simulink model "L03"  (R2020b)
settings: Solver=FixedStepDiscrete  StartTime=0.0  StopTime=50.0  FixedStep=0.01  RelTol=1e-3
undefined symbols (not defined in the file): sigbuilder_block
settings Model: Creator=Nic  LastModifiedBy=Nic

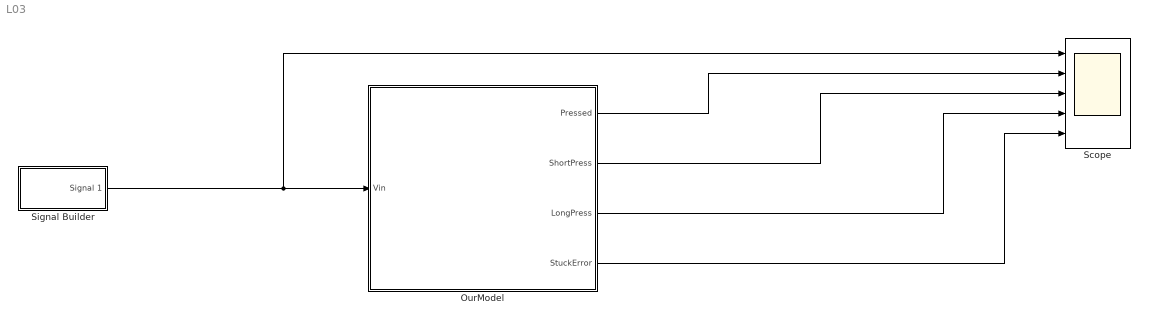
== system L03 ==
  OurModel : Subsystem
  Scope : Scope  NumInputPorts=5
  Signal Builder : Subsystem  Tag=STV Subsys  LoadFcn=sigbuilder_block('load',[173.4 138 748.8 400.2 ]);  StartFcn=sigbuilder_block('start');  StopFcn=sigbuilder_block('stop');  ClipboardFcn=sigbuilder_block('clipboard');  mask(Sigbuilder block){tuvar=[0:10]}
      mask help: Simulink:masks:SigbuilderBlock_MD
      mask init:
      | if ~strcmp(get_param(bdroot(gcbh),'SimulationStatus'),'stopped') tuvar = sigbuilder_block('maskInit'); end
      settings: CopyFcn=sigbuilder_block('copy');  DeleteFcn=sigbuilder_block('delete');  ModelCloseFcn=sigbuilder_block('modelClose');  PreSaveFcn=sigbuilder_block('preSave');  PauseFcn=sigbuilder_block('pause');  ContinueFcn=sigbuilder_block('continue');  NameChangeFcn=sigbuilder_block('namechange');  OpenFcn=sigbuilder_block('open',[173.4 138 550.8 400.2 ]);  CloseFcn=sigbuilder_block('close');
      mask Display: plot(0, 0, 100, 100,[2, 2, 32, 32, 2], [68, 8, 8, 68, 68],[32, 2], [38, 38], [32, 19, 2],[53, 60, 44], [32, 17, 17, 2],[16, 16, 31, 31]);txt = getActiveGroup(gcbh);text(2, 100, txt,'verticalAlignment', 'top');
  wires:
  Signal Builder/1(Signal 1) -> Scope/1, OurModel/1(Vin)
  OurModel/1(Pressed) -> Scope/2
  OurModel/2(ShortPress) -> Scope/3
  OurModel/3(LongPress) -> Scope/4
  OurModel/4(StuckError) -> Scope/5

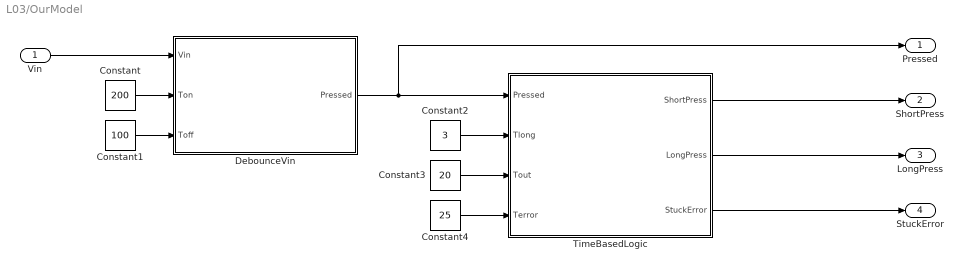
== system L03/OurModel ==
  Vin : Inport
  Constant : Constant  Value=200
  Constant1 : Constant  Value=100
  Constant2 : Constant  Value=3
  Constant3 : Constant  Value=20
  Constant4 : Constant  Value=25
  DebounceVin : Stateflow chart  TreatAsAtomicUnit=on
  TimeBasedLogic : Stateflow chart  TreatAsAtomicUnit=on
  Pressed : Outport
  ShortPress : Outport  Port=2
  LongPress : Outport  Port=3
  StuckError : Outport  Port=4
  wires:
  TimeBasedLogic/3(StuckError) -> StuckError/1
  Constant2/1 -> TimeBasedLogic/2(Tlong)
  DebounceVin/1(Pressed) -> Pressed/1, TimeBasedLogic/1(Pressed)
  Constant/1 -> DebounceVin/2(Ton)
  Vin/1 -> DebounceVin/1(Vin)
  Constant1/1 -> DebounceVin/3(Toff)
  TimeBasedLogic/1(ShortPress) -> ShortPress/1
  Constant3/1 -> TimeBasedLogic/3(Tout)
  TimeBasedLogic/2(LongPress) -> LongPress/1
  Constant4/1 -> TimeBasedLogic/4(Terror)

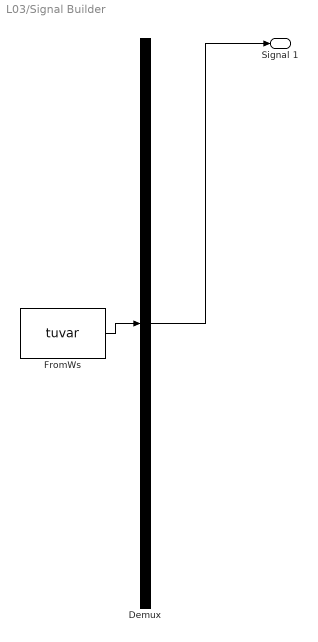
== system L03/Signal Builder ==
  Demux : Demux  Tag=STV Demux  Outputs=1
      settings: DisplayOption=none
  FromWs : FromWorkspace  Tag=STV FromWs  VariableName=tuvar
      SigBuilderData=|
      | common.afterFinalStr = 'Extrapolate'
      | common.sampleTime = 0
      | dataSet.timeRange = [0 50]
      | dataSet.name = 'Group 1'
      | sbobj.Groups.Name = 'Group 1'
      | sbobj.Groups.Signals.Name = 'Signal 1'
      | sbobj.Groups.Signals.XData = [0 1 1 1.14 1.14 2 2 3.5 3.5 3.57 3.57 45.1 45.1 50]
      | sbobj.Groups.Signals.YData = [5 5 0 0 5 5 0 0 5 4.98 0 0 4.96 4.96]
      | sbobj.Groups.TimeRange = [0 50]
  Signal 1 : Outport  Tag=STV Outport
  wires:
  Demux/1 -> Signal 1/1
  FromWs/1 -> Demux/1

== stateflow chart L03/OurModel/TimeBasedLogic ==
  state NOT_PRESSED
    en:
    ShortPress = false;
    LongPress = false;
    StuckError = false;
  state PRESSED
  state LONG
    en:
    ShortPress = false;
    LongPress = true;
    StuckError = false;
  state SHORT
    en:
    ShortPress = true;
    LongPress = false;
    StuckError = false;
  state WAIT_FOR_DEPRESS
    en:
    LongPress = false;
  state STUCK
    en:
    ShortPress = false;
    LongPress = false;
    StuckError = true;
  (default) -> NOT_PRESSED
  (junction 23) -> NOT_PRESSED
  STUCK -> (junction 23) : [Pressed == false]
  (junction 26) -> NOT_PRESSED
  (junction 25) -> (junction 26)
  (junction 21) -> NOT_PRESSED
  WAIT_FOR_DEPRESS -> (junction 21) [order 1] : [Pressed == false]
  NOT_PRESSED -> PRESSED : [Pressed == true]
  PRESSED -> (junction 30) [order 2] : [Pressed == false]
  PRESSED -> LONG [order 1] : [after(Tlong, sec)]
  (junction 30) -> (junction 29)
  (junction 29) -> SHORT
  SHORT -> (junction 25) : [after(Tout, msec)]
  LONG -> WAIT_FOR_DEPRESS : [after(Tout, msec)]
  WAIT_FOR_DEPRESS -> STUCK [order 2] : [after(1000*Terror - 1000*Tlong - Tout, msec)]
  data: Pressed input; Tlong input; Tout input; Terror input; ShortPress output; LongPress output; StuckError output

== stateflow chart L03/OurModel/DebounceVin ==
  state NOT_PRESSED1 [commented out]
    en:
    Pressed = false;
    state NOT_WAIT [commented out]
    state WAIT [commented out]
    NOT_WAIT -> WAIT [commented out] : [Vin < 0.5]
    WAIT -> NOT_WAIT [commented out] : [Vin >= 0.5]
  state NOT_PRESSED
    en:
    Pressed = false;
  state WAIT1
  state WAIT2
  state PRESSED
    en:
    Pressed = true;
  (default) -> NOT_PRESSED1 [commented out]
  (default) -> NOT_PRESSED
  WAIT -> ? [commented out] : [after(Ton, msec)]
  NOT_PRESSED -> WAIT1 : [Vin < 0.5]
  WAIT1 -> NOT_PRESSED [order 1] : [Vin >= 0.5]
  WAIT2 -> NOT_PRESSED [order 2] : [after(Toff, msec)]
  WAIT1 -> PRESSED [order 2] : [after(Ton, msec)]
  PRESSED -> WAIT2 : [Vin >= 4.5]
  WAIT2 -> PRESSED [order 1] : [Vin < 4.5]
  data: Vin input; Ton input; Toff input; Pressed output
